simulink model "RLFactoryEnforceCrash6Opponents"  (R2020a)
settings: Solver=VariableStepAuto  StartTime=0.0  StopTime=60  RelTol=1e-3
undefined symbols (not defined in the file): BLOCKEDTIMER, EPS, getRandomSafeCoord, GoalRange, MAXVELOA, MAXVELOB, MAXVELOC, MAXVELOD, MAXVELOE, MAXVELOF, rl, RLStartX, RLStartY, SAFETYDISTANCEA, SAFETYDISTANCEB, SAFETYDISTANCEC, SAFETYDISTANCED, SAFETYDISTANCEE, SAFETYDISTANCEF, THRESHOLDA, THRESHOLDB, THRESHOLDC, THRESHOLDD, THRESHOLDE, THRESHOLDF, TSA, TSB, TSC, TSD, TSE, TSF, TSRL
libraries: rllib x1
(part 2 of 3)

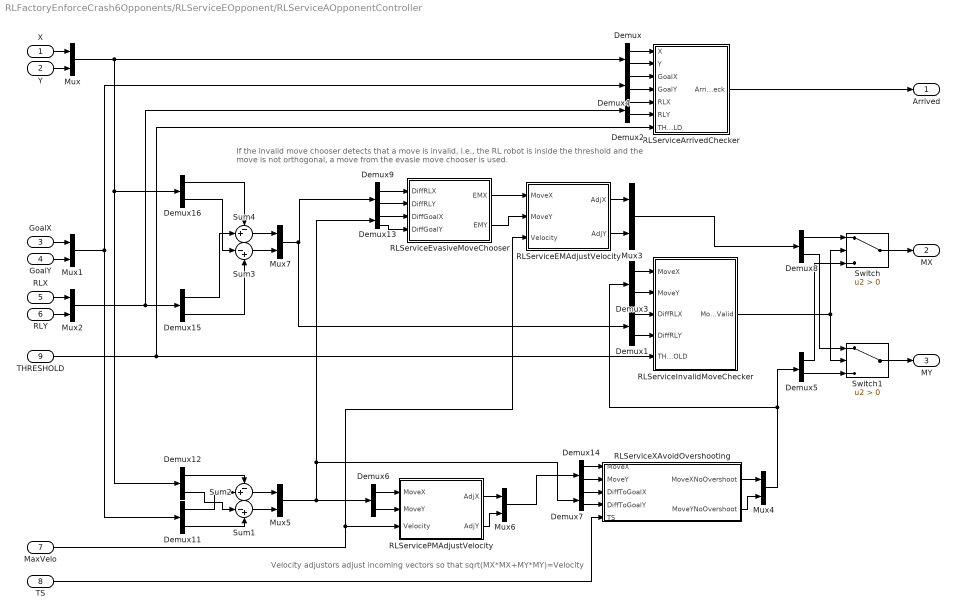
== system RLFactoryEnforceCrash6Opponents/RLServiceEOpponent/RLServiceAOpponentController ==
  note: If the invalid move chooser detects that a move is invalid, i.e.,
      | the RL robot is inside the threshold and the move is not orthogonal, a move from the evasie move chooser is used.
  note: Velocity adjustors adjust incoming vectors so that sqrt(MX*MX+MY*MY)=Velocity
  X : Inport
  Y : Inport  Port=2
  GoalX : Inport  Port=3
  GoalY : Inport  Port=4
  RLX : Inport  Port=5
  RLY : Inport  Port=6
  MaxVelo : Inport  Port=7
  TS : Inport  Port=8
  THRESHOLD : Inport  Port=9
  Demux{,1..9,11..16} (16 alike) : Demux  Outputs=2
  Mux{,1..7} (8 alike) : Mux  Inputs=2
  RLServiceArrivedChecker : Subsystem
  RLServiceEMAdjustVelocity : Subsystem
  RLServiceEvasiveMoveChooser : Subsystem
  RLServiceInvalidMoveChecker : Subsystem
  RLServicePMAdjustVelocity : Subsystem
  RLServiceXAvoidOvershooting : Subsystem
  Sum1 : Sum  Inputs=|-+
  Sum2 : Sum  Inputs=-+|
  Sum3 : Sum  Inputs=|-+
  Sum4 : Sum  Inputs=-+|
  Switch : Switch  Criteria=u2 > Threshold
  Switch1 : Switch  Criteria=u2 > Threshold
  Arrived : Outport
  MX : Outport  Port=2
  MY : Outport  Port=3
  wires:
  GoalX/1 -> Mux1/1
  GoalY/1 -> Mux1/2
  RLServiceArrivedChecker/1(ArrivedCheck) -> Arrived/1
  Demux/1 -> RLServiceArrivedChecker/1(X)
  Demux/2 -> RLServiceArrivedChecker/2(Y)
  Demux4/1 -> RLServiceArrivedChecker/3(GoalX)
  Demux4/2 -> RLServiceArrivedChecker/4(GoalY)
  X/1 -> Mux/1
  Y/1 -> Mux/2
  RLX/1 -> Mux2/1
  RLY/1 -> Mux2/2
  Demux3/1 -> RLServiceInvalidMoveChecker/1(MoveX)
  Demux8/1 -> Switch/1
  Demux5/2 -> Switch1/3
  Demux8/2 -> Switch1/1
  THRESHOLD/1 -> RLServiceArrivedChecker/7(THRESHOLD), RLServiceInvalidMoveChecker/5(THRESHOLD)
  Demux3/2 -> RLServiceInvalidMoveChecker/2(MoveY)
  Demux5/1 -> Switch/3
  RLServiceInvalidMoveChecker/1(MoveInValid) -> Switch/2, Switch1/2
  Switch/1 -> MX/1
  Switch1/1 -> MY/1
  Mux5/1 -> Demux6/1, Demux7/1, Demux13/1
  Demux6/2 -> RLServicePMAdjustVelocity/2(MoveY)
  Mux1/1 -> Demux4/1, Demux11/1
  TS/1 -> RLServiceXAvoidOvershooting/5(TS)
  MaxVelo/1 -> RLServiceEMAdjustVelocity/3(Velocity), RLServicePMAdjustVelocity/3(Velocity)
  RLServicePMAdjustVelocity/1(AdjX) -> Mux6/1
  RLServicePMAdjustVelocity/2(AdjY) -> Mux6/2
  RLServiceEvasiveMoveChooser/1(EMX) -> RLServiceEMAdjustVelocity/1(MoveX)
  RLServiceEvasiveMoveChooser/2(EMY) -> RLServiceEMAdjustVelocity/2(MoveY)
  RLServiceEMAdjustVelocity/1(AdjX) -> Mux3/1
  RLServiceEMAdjustVelocity/2(AdjY) -> Mux3/2
  Mux3/1 -> Demux8/1
  RLServiceXAvoidOvershooting/1(MoveXNoOvershoot) -> Mux4/1
  RLServiceXAvoidOvershooting/2(MoveYNoOvershoot) -> Mux4/2
  Mux4/1 -> Demux5/1, Demux3/1
  Sum2/1 -> Mux5/1
  Sum1/1 -> Mux5/2
  Demux6/1 -> RLServicePMAdjustVelocity/1(MoveX)
  Demux7/1 -> RLServiceXAvoidOvershooting/3(DiffToGoalX)
  Demux7/2 -> RLServiceXAvoidOvershooting/4(DiffToGoalY)
  Demux13/1 -> RLServiceEvasiveMoveChooser/3(DiffGoalX)
  Demux13/2 -> RLServiceEvasiveMoveChooser/4(DiffGoalY)
  Demux11/1 -> Sum2/2
  Demux12/2 -> Sum1/1
  Demux11/2 -> Sum1/2
  Demux12/1 -> Sum2/1
  Demux14/1 -> RLServiceXAvoidOvershooting/1(MoveX)
  Demux14/2 -> RLServiceXAvoidOvershooting/2(MoveY)
  Mux6/1 -> Demux14/1
  Sum3/1 -> Mux7/2
  Demux16/1 -> Sum4/1
  Sum4/1 -> Mux7/1
  Mux/1 -> Demux12/1, Demux16/1, Demux/1
  Mux2/1 -> Demux2/1, Demux15/1
  Demux15/2 -> Sum3/2
  Demux15/1 -> Sum4/2
  Demux16/2 -> Sum3/1
  Demux9/1 -> RLServiceEvasiveMoveChooser/1(DiffRLX)
  Demux9/2 -> RLServiceEvasiveMoveChooser/2(DiffRLY)
  Mux7/1 -> Demux1/1, Demux9/1
  Demux1/1 -> RLServiceInvalidMoveChecker/3(DiffRLX)
  Demux1/2 -> RLServiceInvalidMoveChecker/4(DiffRLY)
  Demux2/2 -> RLServiceArrivedChecker/6(RLY)
  Demux2/1 -> RLServiceArrivedChecker/5(RLX)

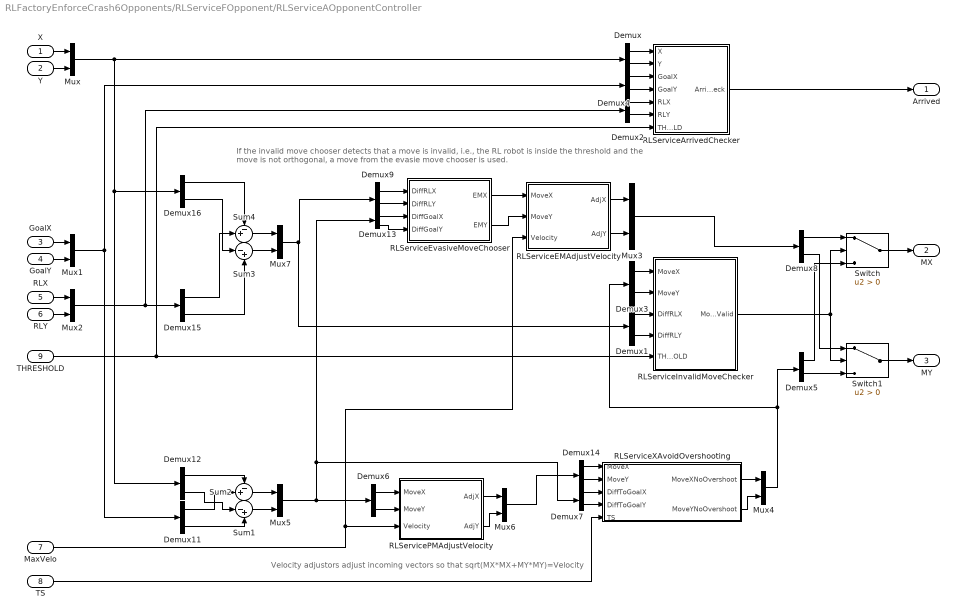
== system RLFactoryEnforceCrash6Opponents/RLServiceFOpponent/RLServiceAOpponentController ==
  note: If the invalid move chooser detects that a move is invalid, i.e.,
      | the RL robot is inside the threshold and the move is not orthogonal, a move from the evasie move chooser is used.
  note: Velocity adjustors adjust incoming vectors so that sqrt(MX*MX+MY*MY)=Velocity
  X : Inport
  Y : Inport  Port=2
  GoalX : Inport  Port=3
  GoalY : Inport  Port=4
  RLX : Inport  Port=5
  RLY : Inport  Port=6
  MaxVelo : Inport  Port=7
  TS : Inport  Port=8
  THRESHOLD : Inport  Port=9
  Demux{,1..9,11..16} (16 alike) : Demux  Outputs=2
  Mux{,1..7} (8 alike) : Mux  Inputs=2
  RLServiceArrivedChecker : Subsystem
  RLServiceEMAdjustVelocity : Subsystem
  RLServiceEvasiveMoveChooser : Subsystem
  RLServiceInvalidMoveChecker : Subsystem
  RLServicePMAdjustVelocity : Subsystem
  RLServiceXAvoidOvershooting : Subsystem
  Sum1 : Sum  Inputs=|-+
  Sum2 : Sum  Inputs=-+|
  Sum3 : Sum  Inputs=|-+
  Sum4 : Sum  Inputs=-+|
  Switch : Switch  Criteria=u2 > Threshold
  Switch1 : Switch  Criteria=u2 > Threshold
  Arrived : Outport
  MX : Outport  Port=2
  MY : Outport  Port=3
  wires:
  GoalX/1 -> Mux1/1
  GoalY/1 -> Mux1/2
  RLServiceArrivedChecker/1(ArrivedCheck) -> Arrived/1
  Demux/1 -> RLServiceArrivedChecker/1(X)
  Demux/2 -> RLServiceArrivedChecker/2(Y)
  Demux4/1 -> RLServiceArrivedChecker/3(GoalX)
  Demux4/2 -> RLServiceArrivedChecker/4(GoalY)
  X/1 -> Mux/1
  Y/1 -> Mux/2
  RLX/1 -> Mux2/1
  RLY/1 -> Mux2/2
  Demux3/1 -> RLServiceInvalidMoveChecker/1(MoveX)
  Demux8/1 -> Switch/1
  Demux5/2 -> Switch1/3
  Demux8/2 -> Switch1/1
  THRESHOLD/1 -> RLServiceArrivedChecker/7(THRESHOLD), RLServiceInvalidMoveChecker/5(THRESHOLD)
  Demux3/2 -> RLServiceInvalidMoveChecker/2(MoveY)
  Demux5/1 -> Switch/3
  RLServiceInvalidMoveChecker/1(MoveInValid) -> Switch/2, Switch1/2
  Switch/1 -> MX/1
  Switch1/1 -> MY/1
  Mux5/1 -> Demux6/1, Demux7/1, Demux13/1
  Demux6/2 -> RLServicePMAdjustVelocity/2(MoveY)
  Mux1/1 -> Demux4/1, Demux11/1
  TS/1 -> RLServiceXAvoidOvershooting/5(TS)
  MaxVelo/1 -> RLServiceEMAdjustVelocity/3(Velocity), RLServicePMAdjustVelocity/3(Velocity)
  RLServicePMAdjustVelocity/1(AdjX) -> Mux6/1
  RLServicePMAdjustVelocity/2(AdjY) -> Mux6/2
  RLServiceEvasiveMoveChooser/1(EMX) -> RLServiceEMAdjustVelocity/1(MoveX)
  RLServiceEvasiveMoveChooser/2(EMY) -> RLServiceEMAdjustVelocity/2(MoveY)
  RLServiceEMAdjustVelocity/1(AdjX) -> Mux3/1
  RLServiceEMAdjustVelocity/2(AdjY) -> Mux3/2
  Mux3/1 -> Demux8/1
  RLServiceXAvoidOvershooting/1(MoveXNoOvershoot) -> Mux4/1
  RLServiceXAvoidOvershooting/2(MoveYNoOvershoot) -> Mux4/2
  Mux4/1 -> Demux5/1, Demux3/1
  Sum2/1 -> Mux5/1
  Sum1/1 -> Mux5/2
  Demux6/1 -> RLServicePMAdjustVelocity/1(MoveX)
  Demux7/1 -> RLServiceXAvoidOvershooting/3(DiffToGoalX)
  Demux7/2 -> RLServiceXAvoidOvershooting/4(DiffToGoalY)
  Demux13/1 -> RLServiceEvasiveMoveChooser/3(DiffGoalX)
  Demux13/2 -> RLServiceEvasiveMoveChooser/4(DiffGoalY)
  Demux11/1 -> Sum2/2
  Demux12/2 -> Sum1/1
  Demux11/2 -> Sum1/2
  Demux12/1 -> Sum2/1
  Demux14/1 -> RLServiceXAvoidOvershooting/1(MoveX)
  Demux14/2 -> RLServiceXAvoidOvershooting/2(MoveY)
  Mux6/1 -> Demux14/1
  Sum3/1 -> Mux7/2
  Demux16/1 -> Sum4/1
  Sum4/1 -> Mux7/1
  Mux/1 -> Demux12/1, Demux16/1, Demux/1
  Mux2/1 -> Demux2/1, Demux15/1
  Demux15/2 -> Sum3/2
  Demux15/1 -> Sum4/2
  Demux16/2 -> Sum3/1
  Demux9/1 -> RLServiceEvasiveMoveChooser/1(DiffRLX)
  Demux9/2 -> RLServiceEvasiveMoveChooser/2(DiffRLY)
  Mux7/1 -> Demux1/1, Demux9/1
  Demux1/1 -> RLServiceInvalidMoveChecker/3(DiffRLX)
  Demux1/2 -> RLServiceInvalidMoveChecker/4(DiffRLY)
  Demux2/2 -> RLServiceArrivedChecker/6(RLY)
  Demux2/1 -> RLServiceArrivedChecker/5(RLX)

== system RLFactoryEnforceCrash6Opponents/RLService6RLRobot/RLService6RLRobotSensor/RLServiceARobotSensorSubsystem ==
  X : Inport
  Y : Inport  Port=2
  OppX : Inport  Port=3
  OppY : Inport  Port=4
  Demux4 : Demux  Outputs=2
  Demux6 : Demux  Outputs=2
  Mux : Mux  Inputs=2
  Mux1 : Mux  Inputs=2
  RLServiceDirectionCalculator : Subsystem
  Sum : Sum  Inputs=-+|
  DiffOppX : Outport
  DiffOppY : Outport  Port=2
  DirOppX : Outport  Port=3
  DirOppY : Outport  Port=4
  wires:
  Mux/1 -> Sum/2, Demux6/1
  Demux6/2 -> RLServiceDirectionCalculator/2(OppY)
  OppX/1 -> Mux/1
  X/1 -> Mux1/1
  Y/1 -> Mux1/2
  Demux6/1 -> RLServiceDirectionCalculator/1(OppX)
  RLServiceDirectionCalculator/1(DirOppX) -> DirOppX/1
  OppY/1 -> Mux/2
  Mux1/1 -> Sum/1
  Sum/1 -> Demux4/1
  RLServiceDirectionCalculator/2(DirOppY) -> DirOppY/1
  Demux4/1 -> DiffOppX/1
  Demux4/2 -> DiffOppY/1

== system RLFactoryEnforceCrash6Opponents/RLService6RLRobot/RLService6RLRobotSensor/RLServiceBRobotSensorSubsystem ==
  X : Inport
  Y : Inport  Port=2
  OppX : Inport  Port=3
  OppY : Inport  Port=4
  Demux4 : Demux  Outputs=2
  Demux6 : Demux  Outputs=2
  Mux : Mux  Inputs=2
  Mux1 : Mux  Inputs=2
  RLServiceDirectionCalculator : Subsystem
  Sum : Sum  Inputs=-+|
  DiffOppX : Outport
  DiffOppY : Outport  Port=2
  DirOppX : Outport  Port=3
  DirOppY : Outport  Port=4
  wires:
  Mux/1 -> Sum/2, Demux6/1
  Demux6/2 -> RLServiceDirectionCalculator/2(OppY)
  OppX/1 -> Mux/1
  X/1 -> Mux1/1
  Y/1 -> Mux1/2
  Demux6/1 -> RLServiceDirectionCalculator/1(OppX)
  RLServiceDirectionCalculator/1(DirOppX) -> DirOppX/1
  OppY/1 -> Mux/2
  Mux1/1 -> Sum/1
  Sum/1 -> Demux4/1
  RLServiceDirectionCalculator/2(DirOppY) -> DirOppY/1
  Demux4/1 -> DiffOppX/1
  Demux4/2 -> DiffOppY/1

== system RLFactoryEnforceCrash6Opponents/RLService6RLRobot/RLService6RLRobotSensor/RLServiceCRobotSensorSubsystem ==
  X : Inport
  Y : Inport  Port=2
  OppX : Inport  Port=3
  OppY : Inport  Port=4
  Demux4 : Demux  Outputs=2
  Demux6 : Demux  Outputs=2
  Mux : Mux  Inputs=2
  Mux1 : Mux  Inputs=2
  RLServiceDirectionCalculator : Subsystem
  Sum : Sum  Inputs=-+|
  DiffOppX : Outport
  DiffOppY : Outport  Port=2
  DirOppX : Outport  Port=3
  DirOppY : Outport  Port=4
  wires:
  Mux/1 -> Sum/2, Demux6/1
  Demux6/2 -> RLServiceDirectionCalculator/2(OppY)
  OppX/1 -> Mux/1
  X/1 -> Mux1/1
  Y/1 -> Mux1/2
  Demux6/1 -> RLServiceDirectionCalculator/1(OppX)
  RLServiceDirectionCalculator/1(DirOppX) -> DirOppX/1
  OppY/1 -> Mux/2
  Mux1/1 -> Sum/1
  Sum/1 -> Demux4/1
  RLServiceDirectionCalculator/2(DirOppY) -> DirOppY/1
  Demux4/1 -> DiffOppX/1
  Demux4/2 -> DiffOppY/1

== system RLFactoryEnforceCrash6Opponents/RLService6RLRobot/RLService6RLRobotSensor/RLServiceDRobotSensorSubsystem ==
  X : Inport
  Y : Inport  Port=2
  OppX : Inport  Port=3
  OppY : Inport  Port=4
  Demux4 : Demux  Outputs=2
  Demux6 : Demux  Outputs=2
  Mux : Mux  Inputs=2
  Mux1 : Mux  Inputs=2
  RLServiceDirectionCalculator : Subsystem
  Sum : Sum  Inputs=-+|
  DiffOppX : Outport
  DiffOppY : Outport  Port=2
  DirOppX : Outport  Port=3
  DirOppY : Outport  Port=4
  wires:
  Mux/1 -> Sum/2, Demux6/1
  Demux6/2 -> RLServiceDirectionCalculator/2(OppY)
  OppX/1 -> Mux/1
  X/1 -> Mux1/1
  Y/1 -> Mux1/2
  Demux6/1 -> RLServiceDirectionCalculator/1(OppX)
  RLServiceDirectionCalculator/1(DirOppX) -> DirOppX/1
  OppY/1 -> Mux/2
  Mux1/1 -> Sum/1
  Sum/1 -> Demux4/1
  RLServiceDirectionCalculator/2(DirOppY) -> DirOppY/1
  Demux4/1 -> DiffOppX/1
  Demux4/2 -> DiffOppY/1

== system RLFactoryEnforceCrash6Opponents/RLService6RLRobot/RLService6RLRobotSensor/RLServiceERobotSensorSubsystem ==
  X : Inport
  Y : Inport  Port=2
  OppX : Inport  Port=3
  OppY : Inport  Port=4
  Demux4 : Demux  Outputs=2
  Demux6 : Demux  Outputs=2
  Mux : Mux  Inputs=2
  Mux1 : Mux  Inputs=2
  RLServiceDirectionCalculator : Subsystem
  Sum : Sum  Inputs=-+|
  DiffOppX : Outport
  DiffOppY : Outport  Port=2
  DirOppX : Outport  Port=3
  DirOppY : Outport  Port=4
  wires:
  Mux/1 -> Sum/2, Demux6/1
  Demux6/2 -> RLServiceDirectionCalculator/2(OppY)
  OppX/1 -> Mux/1
  X/1 -> Mux1/1
  Y/1 -> Mux1/2
  Demux6/1 -> RLServiceDirectionCalculator/1(OppX)
  RLServiceDirectionCalculator/1(DirOppX) -> DirOppX/1
  OppY/1 -> Mux/2
  Mux1/1 -> Sum/1
  Sum/1 -> Demux4/1
  RLServiceDirectionCalculator/2(DirOppY) -> DirOppY/1
  Demux4/1 -> DiffOppX/1
  Demux4/2 -> DiffOppY/1

== system RLFactoryEnforceCrash6Opponents/RLService6RLRobot/RLService6RLRobotSensor/RLServiceFRobotSensorSubsystem ==
  X : Inport
  Y : Inport  Port=2
  OppX : Inport  Port=3
  OppY : Inport  Port=4
  Demux4 : Demux  Outputs=2
  Demux6 : Demux  Outputs=2
  Mux : Mux  Inputs=2
  Mux1 : Mux  Inputs=2
  RLServiceDirectionCalculator : Subsystem
  Sum : Sum  Inputs=-+|
  DiffOppX : Outport
  DiffOppY : Outport  Port=2
  DirOppX : Outport  Port=3
  DirOppY : Outport  Port=4
  wires:
  Mux/1 -> Sum/2, Demux6/1
  Demux6/2 -> RLServiceDirectionCalculator/2(OppY)
  OppX/1 -> Mux/1
  X/1 -> Mux1/1
  Y/1 -> Mux1/2
  Demux6/1 -> RLServiceDirectionCalculator/1(OppX)
  RLServiceDirectionCalculator/1(DirOppX) -> DirOppX/1
  OppY/1 -> Mux/2
  Mux1/1 -> Sum/1
  Sum/1 -> Demux4/1
  RLServiceDirectionCalculator/2(DirOppY) -> DirOppY/1
  Demux4/1 -> DiffOppX/1
  Demux4/2 -> DiffOppY/1

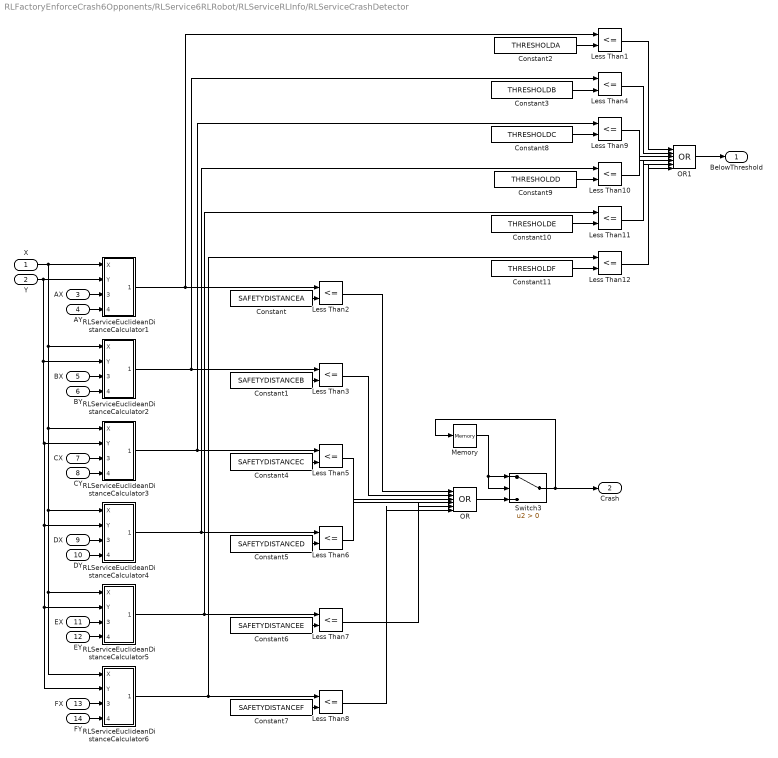
== system RLFactoryEnforceCrash6Opponents/RLService6RLRobot/RLServiceRLInfo/RLServiceCrashDetector ==
  X : Inport
  Y : Inport  Port=2
  AX : Inport  Port=3
  AY : Inport  Port=4
  BX : Inport  Port=5
  BY : Inport  Port=6
  CX : Inport  Port=7
  CY : Inport  Port=8
  DX : Inport  Port=9
  DY : Inport  Port=10
  EX : Inport  Port=11
  EY : Inport  Port=12
  FX : Inport  Port=13
  FY : Inport  Port=14
  Constant : Constant  Value=SAFETYDISTANCEA
  Constant1 : Constant  Value=SAFETYDISTANCEB
  Constant10 : Constant  Value=THRESHOLDE
  Constant11 : Constant  Value=THRESHOLDF
  Constant2 : Constant  Value=THRESHOLDA
  Constant3 : Constant  Value=THRESHOLDB
  Constant4 : Constant  Value=SAFETYDISTANCEC
  Constant5 : Constant  Value=SAFETYDISTANCED
  Constant6 : Constant  Value=SAFETYDISTANCEE
  Constant7 : Constant  Value=SAFETYDISTANCEF
  Constant8 : Constant  Value=THRESHOLDC
  Constant9 : Constant  Value=THRESHOLDD
  Less Than{1..12} (12 alike) : RelationalOperator  Operator=<=  OutDataTypeStr=boolean  RndMeth=Simplest
  Memory : Memory
  OR : Logic  Operator=OR  Inputs=6  IconShape=distinctive  AllPortsSameDT=off  OutDataTypeStr=boolean
  OR1 : Logic  Operator=OR  Inputs=6  IconShape=distinctive  AllPortsSameDT=off  OutDataTypeStr=boolean
  RLServiceEuclideanDistanceCalculator1 : Subsystem
  RLServiceEuclideanDistanceCalculator2 : Subsystem
  RLServiceEuclideanDistanceCalculator3 : Subsystem
  RLServiceEuclideanDistanceCalculator4 : Subsystem
  RLServiceEuclideanDistanceCalculator5 : Subsystem
  RLServiceEuclideanDistanceCalculator6 : Subsystem
  Switch3 : Switch  Criteria=u2 > Threshold
  BelowThreshold : Outport
  Crash : Outport  Port=2
  wires:
  AX/1 -> RLServiceEuclideanDistanceCalculator1/3(XOpp)
  Less Than2/1 -> OR/1
  Memory/1 -> Switch3/2, Switch3/1
  Constant/1 -> Less Than2/2
  AY/1 -> RLServiceEuclideanDistanceCalculator1/4(YOpp)
  OR/1 -> Switch3/3
  Constant1/1 -> Less Than3/2
  BY/1 -> RLServiceEuclideanDistanceCalculator2/4(YOpp)
  Less Than3/1 -> OR/2
  BX/1 -> RLServiceEuclideanDistanceCalculator2/3(XOpp)
  Switch3/1 -> Crash/1, Memory/1
  Constant2/1 -> Less Than1/2
  RLServiceEuclideanDistanceCalculator1/1(Dist) -> Less Than2/1, Less Than1/1
  Constant3/1 -> Less Than4/2
  RLServiceEuclideanDistanceCalculator2/1(Dist) -> Less Than4/1, Less Than3/1
  Less Than1/1 -> OR1/1
  Less Than4/1 -> OR1/2
  OR1/1 -> BelowThreshold/1
  DY/1 -> RLServiceEuclideanDistanceCalculator4/4(YOpp)
  Less Than5/1 -> OR/3
  Constant5/1 -> Less Than6/2
  Constant4/1 -> Less Than5/2
  RLServiceEuclideanDistanceCalculator3/1(Dist) -> Less Than9/1, Less Than5/1
  Less Than6/1 -> OR/4
  DX/1 -> RLServiceEuclideanDistanceCalculator4/3(XOpp)
  CX/1 -> RLServiceEuclideanDistanceCalculator3/3(XOpp)
  RLServiceEuclideanDistanceCalculator4/1(Dist) -> Less Than10/1, Less Than6/1
  CY/1 -> RLServiceEuclideanDistanceCalculator3/4(YOpp)
  EX/1 -> RLServiceEuclideanDistanceCalculator5/3(XOpp)
  EY/1 -> RLServiceEuclideanDistanceCalculator5/4(YOpp)
  RLServiceEuclideanDistanceCalculator5/1(Dist) -> Less Than7/1, Less Than11/1
  Constant6/1 -> Less Than7/2
  FY/1 -> RLServiceEuclideanDistanceCalculator6/4(YOpp)
  Constant7/1 -> Less Than8/2
  Y/1 -> RLServiceEuclideanDistanceCalculator6/2(Y), RLServiceEuclideanDistanceCalculator5/2(Y), RLServiceEuclideanDistanceCalculator4/2(Y), RLServiceEuclideanDistanceCalculator3/2(Y), RLServiceEuclideanDistanceCalculator2/2(Y), RLServiceEuclideanDistanceCalculator1/2(Y)
  X/1 -> RLServiceEuclideanDistanceCalculator1/1(X), RLServiceEuclideanDistanceCalculator6/1(X), RLServiceEuclideanDistanceCalculator5/1(X), RLServiceEuclideanDistanceCalculator4/1(X), RLServiceEuclideanDistanceCalculator3/1(X), RLServiceEuclideanDistanceCalculator2/1(X)
  FX/1 -> RLServiceEuclideanDistanceCalculator6/3(XOpp)
  RLServiceEuclideanDistanceCalculator6/1(Dist) -> Less Than8/1, Less Than12/1
  Less Than7/1 -> OR/5
  Less Than8/1 -> OR/6
  Constant8/1 -> Less Than9/2
  Less Than9/1 -> OR1/3
  Less Than11/1 -> OR1/5
  Less Than10/1 -> OR1/4
  Constant10/1 -> Less Than11/2
  Constant9/1 -> Less Than10/2
  Less Than12/1 -> OR1/6
  Constant11/1 -> Less Than12/2

== system RLFactoryEnforceCrash6Opponents/RLService6RLRobot/RLServiceRLInfo/RLServiceGoalTracker ==
  X : Inport
  Y : Inport  Port=2
  GoalX : Inport  Port=3
  GoalY : Inport  Port=4
  Constant1 : Constant
  Constant5 : Constant  Value=0.5
  Constant7 : Constant  Value=0
  Less Than1 : RelationalOperator  Operator=<  OutDataTypeStr=boolean  RndMeth=Simplest
  RLServiceEuclideanDistanceCalculator : Subsystem
  Switch : Switch  Criteria=u2 > Threshold
  Dist : Outport
  Arrived : Outport  Port=2
  wires:
  Constant7/1 -> Switch/3
  GoalX/1 -> RLServiceEuclideanDistanceCalculator/3(GoalX)
  Y/1 -> RLServiceEuclideanDistanceCalculator/2(Y)
  RLServiceEuclideanDistanceCalculator/1(DistGoal) -> Dist/1, Less Than1/1
  Constant1/1 -> Switch/1
  Switch/1 -> Arrived/1
  Less Than1/1 -> Switch/2
  X/1 -> RLServiceEuclideanDistanceCalculator/1(X)
  GoalY/1 -> RLServiceEuclideanDistanceCalculator/4(GoalY)
  Constant5/1 -> Less Than1/2

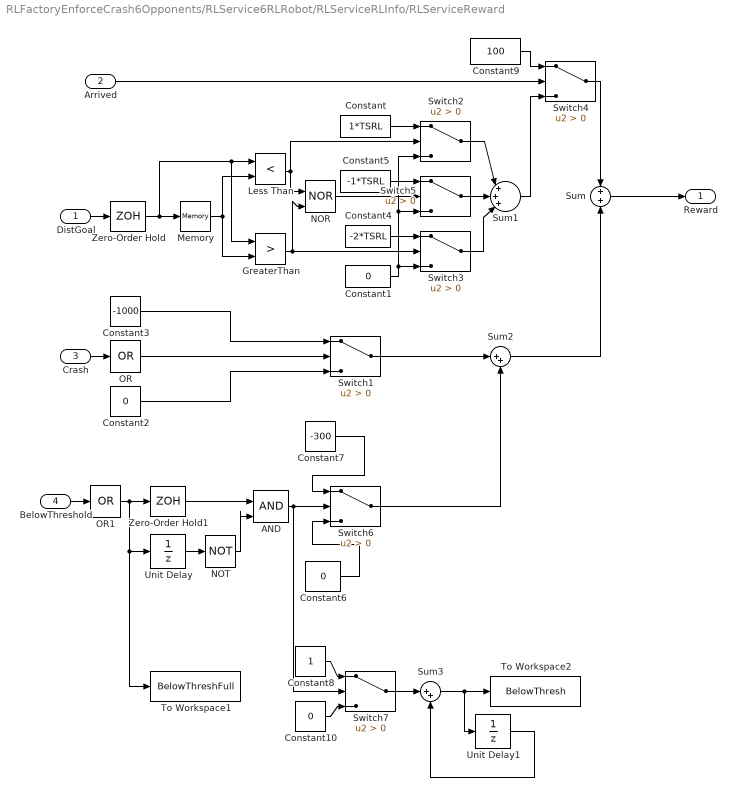
== system RLFactoryEnforceCrash6Opponents/RLService6RLRobot/RLServiceRLInfo/RLServiceReward ==
  DistGoal : Inport
  Arrived : Inport  Port=2
  Crash : Inport  Port=3
  BelowThreshold : Inport  Port=4
  AND : Logic  IconShape=distinctive  AllPortsSameDT=off  OutDataTypeStr=boolean
  Constant : Constant  Value=1*TSRL
  Constant{1..2,6,10} (4 alike) : Constant  Value=0
  Constant3 : Constant  Value=-1000  VectorParams1D=off
  Constant4 : Constant  Value=-2*TSRL
  Constant5 : Constant  Value=-1*TSRL
  Constant7 : Constant  Value=-300  VectorParams1D=off
  Constant8 : Constant
  Constant9 : Constant  Value=100
  GreaterThan : RelationalOperator  Operator=>  OutDataTypeStr=boolean  RndMeth=Simplest
  Less Than : RelationalOperator  Operator=<  OutDataTypeStr=boolean  RndMeth=Simplest
  Memory : Memory
  NOR : Logic  Operator=NOR  IconShape=distinctive  AllPortsSameDT=off  OutDataTypeStr=boolean
  NOT : Logic  Operator=NOT  IconShape=distinctive  AllPortsSameDT=off  OutDataTypeStr=boolean
  OR : Logic  Operator=OR  Inputs=1  IconShape=distinctive  AllPortsSameDT=off  OutDataTypeStr=boolean
  OR1 : Logic  Operator=OR  Inputs=1  IconShape=distinctive  AllPortsSameDT=off  OutDataTypeStr=boolean
  Sum : Sum
  Sum1 : Sum  Inputs=|+++|
  Sum2 : Sum  Inputs=|++
  Sum3 : Sum  Inputs=|++
  Switch{1..7} (7 alike) : Switch  Criteria=u2 > Threshold
  To Workspace1 : ToWorkspace  VariableName=BelowThreshFull  SampleTime=TSRL
  To Workspace2 : ToWorkspace  VariableName=BelowThresh  SampleTime=TSRL
      settings: MaxDataPoints=1
  Unit Delay : UnitDelay  SampleTime=TSRL  HasFrameUpgradeWarning=on
  Unit Delay1 : UnitDelay  SampleTime=TSRL  HasFrameUpgradeWarning=on
  Zero-Order Hold : ZeroOrderHold  SampleTime=TSRL
  Zero-Order Hold1 : ZeroOrderHold  SampleTime=TSRL
  Reward : Outport
  wires:
  Sum/1 -> Reward/1
  Constant2/1 -> Switch1/3
  Constant3/1 -> Switch1/1
  Sum2/1 -> Sum/2
  DistGoal/1 -> Zero-Order Hold/1
  Memory/1 -> GreaterThan/2, Less Than/2
  Switch4/1 -> Sum/1
  Constant9/1 -> Switch4/1
  Switch2/1 -> Sum1/1
  Arrived/1 -> Switch4/2
  OR/1 -> Switch1/2
  Less Than/1 -> NOR/1, Switch2/2
  Constant/1 -> Switch2/1
  Constant1/1 -> Switch2/3, Switch5/3, Switch3/3
  GreaterThan/1 -> NOR/2, Switch3/2
  Constant4/1 -> Switch3/1
  Sum1/1 -> Switch4/3
  Switch3/1 -> Sum1/3
  NOR/1 -> Switch5/2
  Constant5/1 -> Switch5/1
  Switch5/1 -> Sum1/2
  Zero-Order Hold/1 -> Memory/1, GreaterThan/1, Less Than/1
  Crash/1 -> OR/1
  OR1/1 -> Zero-Order Hold1/1, To Workspace1/1, Unit Delay/1
  Constant7/1 -> Switch6/1
  BelowThreshold/1 -> OR1/1
  Constant6/1 -> Switch6/3
  Switch6/1 -> Sum2/2
  Switch1/1 -> Sum2/1
  Unit Delay/1 -> NOT/1
  NOT/1 -> AND/2
  Sum3/1 -> To Workspace2/1, Unit Delay1/1
  Zero-Order Hold1/1 -> AND/1
  Unit Delay1/1 -> Sum3/2
  Switch7/1 -> Sum3/1
  Constant8/1 -> Switch7/1
  Constant10/1 -> Switch7/3
  AND/1 -> Switch7/2, Switch6/2

== system RLFactoryEnforceCrash6Opponents/RLService6RLRobot/RLServiceRLMotorControl/RLServiceRLAdjustVelocity ==
  MoveX : Inport
  MoveY : Inport  Port=2
  Velocity : Inport  Port=3
  Constant : Constant
  Demux1 : Demux  Outputs=2
  Divide : Product  Inputs=*/
  Divide1 : Product  Inputs=*/
  Mux : Mux  Inputs=2
  Product : Product
  Product3 : Product
  Sqrt1 : Sqrt  SaturateOnIntegerOverflow=on
  Square : Math  Operator=square  SaturateOnIntegerOverflow=on
  Square1 : Math  Operator=square  SaturateOnIntegerOverflow=on
  Sum : Sum  Inputs=+|+
  Switch : Switch  Criteria=u2 > Threshold
  AdjMX : Outport
  AdjMY : Outport  Port=2
  wires:
  Product/1 -> AdjMX/1
  MoveY/1 -> Square1/1, Mux/2
  Mux/1 -> Demux1/1
  Divide1/1 -> Product3/1
  Constant/1 -> Switch/3
  Square1/1 -> Sum/2
  Switch/1 -> Divide1/2, Divide/2
  Velocity/1 -> Product/2, Product3/2
  Sum/1 -> Sqrt1/1
  Square/1 -> Sum/1
  Sqrt1/1 -> Switch/2, Switch/1
  Product3/1 -> AdjMY/1
  Demux1/2 -> Divide1/1
  MoveX/1 -> Square/1, Mux/1
  Demux1/1 -> Divide/1
  Divide/1 -> Product/1

== system RLFactoryEnforceCrash6Opponents/RLServiceAOpponent/RLServiceAOpponentController/RLServiceArrivedChecker ==
  X : Inport
  Y : Inport  Port=2
  GoalX : Inport  Port=3
  GoalY : Inport  Port=4
  RLX : Inport  Port=5
  RLY : Inport  Port=6
  THRESHOLD : Inport  Port=7
  Constant1 : Constant
  Constant3 : Constant
  Constant4 : Constant  Value=0
  Constant5 : Constant  Value=0
  Constant6 : Constant
  Constant8 : Constant  Value=-BLOCKEDTIMER
  Integrator : Integrator  LimitOutput=on  UpperSaturationLimit=BLOCKEDTIMER  LowerSaturationLimit=0
  RLServiceEuclideanDistanceCalculator1 : Subsystem
  RLServiceEuclideanDistanceCalculator2 : Subsystem
  Sum : Sum  Inputs=|++
  Sum1 : Sum  Inputs=+-|
  Switch1 : Switch  Criteria=u2 > Threshold  Threshold=0.5
  Switch3 : Switch  Threshold=BLOCKEDTIMER
  Switch4 : Switch  Criteria=u2 > Threshold
  ArrivedCheck : Outport
  wires:
  RLServiceEuclideanDistanceCalculator1/1(DistToGoal) -> Switch1/2
  X/1 -> RLServiceEuclideanDistanceCalculator1/1(X)
  Switch1/1 -> Sum/1
  Constant3/1 -> Switch1/3
  Y/1 -> RLServiceEuclideanDistanceCalculator1/2(Y)
  Constant4/1 -> Switch1/1
  Sum/1 -> ArrivedCheck/1
  Switch3/1 -> Sum/2
  Integrator/1 -> Switch3/2
  Constant5/1 -> Switch3/3
  RLX/1 -> RLServiceEuclideanDistanceCalculator2/1(X)
  RLY/1 -> RLServiceEuclideanDistanceCalculator2/2(Y)
  GoalX/1 -> RLServiceEuclideanDistanceCalculator2/3(GoalX), RLServiceEuclideanDistanceCalculator1/3(GoalX)
  GoalY/1 -> RLServiceEuclideanDistanceCalculator2/4(GoalY), RLServiceEuclideanDistanceCalculator1/4(GoalY)
  RLServiceEuclideanDistanceCalculator2/1(OppDistToGoal) -> Sum1/1
  Constant8/1 -> Switch4/1
  Constant6/1 -> Switch4/3
  THRESHOLD/1 -> Sum1/2
  Sum1/1 -> Switch4/2
  Switch4/1 -> Integrator/1
  Constant1/1 -> Switch3/1

== system RLFactoryEnforceCrash6Opponents/RLServiceAOpponent/RLServiceAOpponentController/RLServiceEMAdjustVelocity ==
  MoveX : Inport
  MoveY : Inport  Port=2
  Velocity : Inport  Port=3
  Constant : Constant
  Demux1 : Demux  Outputs=2
  Divide : Product  Inputs=*/
  Divide1 : Product  Inputs=*/
  Mux : Mux  Inputs=2
  Product : Product
  Product3 : Product
  Sqrt1 : Sqrt  SaturateOnIntegerOverflow=on
  Square : Math  Operator=square  SaturateOnIntegerOverflow=on
  Square1 : Math  Operator=square  SaturateOnIntegerOverflow=on
  Sum : Sum  Inputs=+|+
  Switch : Switch  Criteria=u2 > Threshold
  AdjX : Outport
  AdjY : Outport  Port=2
  wires:
  Product/1 -> AdjX/1
  MoveY/1 -> Square1/1, Mux/2
  Mux/1 -> Demux1/1
  Divide1/1 -> Product3/1
  Constant/1 -> Switch/3
  Square1/1 -> Sum/2
  Switch/1 -> Divide1/2, Divide/2
  Velocity/1 -> Product/2, Product3/2
  Sum/1 -> Sqrt1/1
  Square/1 -> Sum/1
  Sqrt1/1 -> Switch/2, Switch/1
  Product3/1 -> AdjY/1
  Demux1/2 -> Divide1/1
  MoveX/1 -> Square/1, Mux/1
  Demux1/1 -> Divide/1
  Divide/1 -> Product/1

== system RLFactoryEnforceCrash6Opponents/RLServiceAOpponent/RLServiceAOpponentController/RLServiceEvasiveMoveChooser ==
  DiffRLX : Inport
  DiffRLY : Inport  Port=2
  DiffGoalX : Inport  Port=3
  DiffGoalY : Inport  Port=4
  Abs : Abs
  Abs1 : Abs
  Demux{,2..4} (4 alike) : Demux  Outputs=2
  Gain : Gain  Gain=-1
  Gain1 : Gain  Gain=-1
  Mux1 : Mux  Inputs=2
  Mux2 : Mux  Inputs=2
  Mux3 : Mux  Inputs=2
  Sqrt : Sqrt  SaturateOnIntegerOverflow=on
  Sqrt1 : Sqrt  SaturateOnIntegerOverflow=on
  Sum{,1..2,5} (4 alike) : Sum  Inputs=+|+
  Sum6 : Sum  Inputs=+|-
  Switch : Switch  Criteria=u2 > Threshold
  Switch1 : Switch  Criteria=u2 > Threshold
  EMX : Outport
  EMY : Outport  Port=2
  wires:
  Gain/1 -> Mux1/1
  DiffRLX/1 -> Gain1/1, Mux1/2
  Gain1/1 -> Mux2/2
  DiffGoalX/1 -> Mux3/1
  DiffGoalY/1 -> Mux3/2
  Mux3/1 -> Sum/2, Sum1/2
  Mux2/1 -> Sum/1, Demux4/1
  Mux1/1 -> Demux3/1, Sum1/1
  Sum1/1 -> Abs/1
  Sum/1 -> Abs1/1
  Abs1/1 -> Demux/1
  Demux/1 -> Sum2/1
  Demux/2 -> Sum2/2
  Demux2/2 -> Sum5/2
  Demux2/1 -> Sum5/1
  Abs/1 -> Demux2/1
  Sum5/1 -> Sqrt/1
  Sum2/1 -> Sqrt1/1
  Sqrt/1 -> Sum6/1
  Sqrt1/1 -> Sum6/2
  Sum6/1 -> Switch/2, Switch1/2
  Demux3/1 -> Switch/1
  Demux3/2 -> Switch1/1
  Demux4/1 -> Switch/3
  Demux4/2 -> Switch1/3
  Switch/1 -> EMX/1
  Switch1/1 -> EMY/1
  DiffRLY/1 -> Mux2/1, Gain/1

== system RLFactoryEnforceCrash6Opponents/RLServiceAOpponent/RLServiceAOpponentController/RLServiceInvalidMoveChecker ==
  MoveX : Inport
  MoveY : Inport  Port=2
  DiffRLX : Inport  Port=3
  DiffRLY : Inport  Port=4
  THRESHOLD : Inport  Port=5
  Constant5 : Constant
  Constant6 : Constant  Value=0
  Constant7 : Constant  Value=0
  Constant8 : Constant
  Constant9 : Constant
  Product : Product
  Product1 : Product
  Square : Math  Operator=square  SaturateOnIntegerOverflow=on
  Square Root : Sqrt  SaturateOnIntegerOverflow=on
  Square1 : Math  Operator=square  SaturateOnIntegerOverflow=on
  Sum : Sum  Inputs=+|-
  Sum1 : Sum
  Sum5 : Sum  Inputs=+|+
  Sum6 : Sum  Inputs=+|-|+
  Switch1 : Switch  Criteria=u2 > Threshold
  Switch3 : Switch  Criteria=u2 > Threshold
  MoveInValid : Outport
  wires:
  Product1/1 -> Sum5/2
  Sum5/1 -> Switch3/2
  Product/1 -> Sum5/1
  Sum6/1 -> MoveInValid/1
  Switch3/1 -> Sum6/1
  Constant9/1 -> Switch3/1
  MoveY/1 -> Product1/1
  MoveX/1 -> Product/1
  Constant8/1 -> Sum6/2
  Constant7/1 -> Switch3/3
  THRESHOLD/1 -> Sum/2
  Sum/1 -> Switch1/2
  Constant5/1 -> Switch1/3
  Constant6/1 -> Switch1/1
  Switch1/1 -> Sum6/3
  DiffRLY/1 -> Square1/1, Product1/2
  DiffRLX/1 -> Product/2, Square/1
  Square1/1 -> Sum1/2
  Sum1/1 -> Square Root/1
  Square/1 -> Sum1/1
  Square Root/1 -> Sum/1

== system RLFactoryEnforceCrash6Opponents/RLServiceAOpponent/RLServiceAOpponentController/RLServicePMAdjustVelocity ==
  MoveX : Inport
  MoveY : Inport  Port=2
  Velocity : Inport  Port=3
  Constant : Constant
  Demux1 : Demux  Outputs=2
  Divide : Product  Inputs=*/
  Divide1 : Product  Inputs=*/
  Mux : Mux  Inputs=2
  Product : Product
  Product3 : Product
  Sqrt1 : Sqrt  SaturateOnIntegerOverflow=on
  Square : Math  Operator=square  SaturateOnIntegerOverflow=on
  Square1 : Math  Operator=square  SaturateOnIntegerOverflow=on
  Sum : Sum  Inputs=+|+
  Switch : Switch  Criteria=u2 > Threshold
  AdjX : Outport
  AdjY : Outport  Port=2
  wires:
  Velocity/1 -> Product/2, Product3/2
  MoveX/1 -> Square/1, Mux/1
  MoveY/1 -> Square1/1, Mux/2
  Divide1/1 -> Product3/1
  Divide/1 -> Product/1
  Switch/1 -> Divide1/2, Divide/2
  Constant/1 -> Switch/3
  Mux/1 -> Demux1/1
  Demux1/2 -> Divide1/1
  Square1/1 -> Sum/2
  Sum/1 -> Sqrt1/1
  Demux1/1 -> Divide/1
  Product/1 -> AdjX/1
  Sqrt1/1 -> Switch/2, Switch/1
  Product3/1 -> AdjY/1
  Square/1 -> Sum/1

== system RLFactoryEnforceCrash6Opponents/RLServiceAOpponent/RLServiceAOpponentController/RLServiceXAvoidOvershooting ==
  MoveX : Inport
  MoveY : Inport  Port=2
  DiffToGoalX : Inport  Port=3
  DiffToGoalY : Inport  Port=4
  TS : Inport  Port=5
  Abs{1..4} (4 alike) : Abs
  Divide : Product  Inputs=*/
  Divide1 : Product  Inputs=*/
  Product : Product
  Product1 : Product
  Sum1 : Sum  Inputs=-|+
  Sum2 : Sum  Inputs=-|+
  Switch : Switch  Criteria=u2 > Threshold
  Switch1 : Switch  Criteria=u2 > Threshold
  MoveXNoOvershoot : Outport
  MoveYNoOvershoot : Outport  Port=2
  wires:
  Abs1/1 -> Sum1/2
  Switch/1 -> MoveXNoOvershoot/1
  Product/1 -> Abs2/1
  Abs2/1 -> Sum1/1
  DiffToGoalX/1 -> Divide/1, Abs1/1
  Sum1/1 -> Switch/2
  MoveX/1 -> Product/1, Switch/1
  Divide/1 -> Switch/3
  MoveY/1 -> Product1/1, Switch1/1
  Sum2/1 -> Switch1/2
  Abs4/1 -> Sum2/1
  Product1/1 -> Abs4/1
  Divide1/1 -> Switch1/3
  TS/1 -> Divide1/2, Product1/2, Divide/2, Product/2
  Abs3/1 -> Sum2/2
  Switch1/1 -> MoveYNoOvershoot/1
  DiffToGoalY/1 -> Divide1/1, Abs3/1

== system RLFactoryEnforceCrash6Opponents/RLServiceBOpponent/RLServiceAOpponentController/RLServiceArrivedChecker ==
  X : Inport
  Y : Inport  Port=2
  GoalX : Inport  Port=3
  GoalY : Inport  Port=4
  RLX : Inport  Port=5
  RLY : Inport  Port=6
  THRESHOLD : Inport  Port=7
  Constant1 : Constant
  Constant3 : Constant
  Constant4 : Constant  Value=0
  Constant5 : Constant  Value=0
  Constant6 : Constant
  Constant8 : Constant  Value=-BLOCKEDTIMER
  Integrator : Integrator  LimitOutput=on  UpperSaturationLimit=BLOCKEDTIMER  LowerSaturationLimit=0
  RLServiceEuclideanDistanceCalculator1 : Subsystem
  RLServiceEuclideanDistanceCalculator2 : Subsystem
  Sum : Sum  Inputs=|++
  Sum1 : Sum  Inputs=+-|
  Switch1 : Switch  Criteria=u2 > Threshold  Threshold=0.5
  Switch3 : Switch  Threshold=BLOCKEDTIMER
  Switch4 : Switch  Criteria=u2 > Threshold
  ArrivedCheck : Outport
  wires:
  RLServiceEuclideanDistanceCalculator1/1(DistToGoal) -> Switch1/2
  X/1 -> RLServiceEuclideanDistanceCalculator1/1(X)
  Switch1/1 -> Sum/1
  Constant3/1 -> Switch1/3
  Y/1 -> RLServiceEuclideanDistanceCalculator1/2(Y)
  Constant4/1 -> Switch1/1
  Sum/1 -> ArrivedCheck/1
  Switch3/1 -> Sum/2
  Integrator/1 -> Switch3/2
  Constant5/1 -> Switch3/3
  RLX/1 -> RLServiceEuclideanDistanceCalculator2/1(X)
  RLY/1 -> RLServiceEuclideanDistanceCalculator2/2(Y)
  GoalX/1 -> RLServiceEuclideanDistanceCalculator2/3(GoalX), RLServiceEuclideanDistanceCalculator1/3(GoalX)
  GoalY/1 -> RLServiceEuclideanDistanceCalculator2/4(GoalY), RLServiceEuclideanDistanceCalculator1/4(GoalY)
  RLServiceEuclideanDistanceCalculator2/1(OppDistToGoal) -> Sum1/1
  Constant8/1 -> Switch4/1
  Constant6/1 -> Switch4/3
  THRESHOLD/1 -> Sum1/2
  Sum1/1 -> Switch4/2
  Switch4/1 -> Integrator/1
  Constant1/1 -> Switch3/1

== system RLFactoryEnforceCrash6Opponents/RLServiceBOpponent/RLServiceAOpponentController/RLServiceEMAdjustVelocity ==
  MoveX : Inport
  MoveY : Inport  Port=2
  Velocity : Inport  Port=3
  Constant : Constant
  Demux1 : Demux  Outputs=2
  Divide : Product  Inputs=*/
  Divide1 : Product  Inputs=*/
  Mux : Mux  Inputs=2
  Product : Product
  Product3 : Product
  Sqrt1 : Sqrt  SaturateOnIntegerOverflow=on
  Square : Math  Operator=square  SaturateOnIntegerOverflow=on
  Square1 : Math  Operator=square  SaturateOnIntegerOverflow=on
  Sum : Sum  Inputs=+|+
  Switch : Switch  Criteria=u2 > Threshold
  AdjX : Outport
  AdjY : Outport  Port=2
  wires:
  Product/1 -> AdjX/1
  MoveY/1 -> Square1/1, Mux/2
  Mux/1 -> Demux1/1
  Divide1/1 -> Product3/1
  Constant/1 -> Switch/3
  Square1/1 -> Sum/2
  Switch/1 -> Divide1/2, Divide/2
  Velocity/1 -> Product/2, Product3/2
  Sum/1 -> Sqrt1/1
  Square/1 -> Sum/1
  Sqrt1/1 -> Switch/2, Switch/1
  Product3/1 -> AdjY/1
  Demux1/2 -> Divide1/1
  MoveX/1 -> Square/1, Mux/1
  Demux1/1 -> Divide/1
  Divide/1 -> Product/1

== system RLFactoryEnforceCrash6Opponents/RLServiceBOpponent/RLServiceAOpponentController/RLServiceEvasiveMoveChooser ==
  DiffRLX : Inport
  DiffRLY : Inport  Port=2
  DiffGoalX : Inport  Port=3
  DiffGoalY : Inport  Port=4
  Abs : Abs
  Abs1 : Abs
  Demux{,2..4} (4 alike) : Demux  Outputs=2
  Gain : Gain  Gain=-1
  Gain1 : Gain  Gain=-1
  Mux1 : Mux  Inputs=2
  Mux2 : Mux  Inputs=2
  Mux3 : Mux  Inputs=2
  Sqrt : Sqrt  SaturateOnIntegerOverflow=on
  Sqrt1 : Sqrt  SaturateOnIntegerOverflow=on
  Sum{,1..2,5} (4 alike) : Sum  Inputs=+|+
  Sum6 : Sum  Inputs=+|-
  Switch : Switch  Criteria=u2 > Threshold
  Switch1 : Switch  Criteria=u2 > Threshold
  EMX : Outport
  EMY : Outport  Port=2
  wires:
  Gain/1 -> Mux1/1
  DiffRLX/1 -> Gain1/1, Mux1/2
  Gain1/1 -> Mux2/2
  DiffGoalX/1 -> Mux3/1
  DiffGoalY/1 -> Mux3/2
  Mux3/1 -> Sum/2, Sum1/2
  Mux2/1 -> Sum/1, Demux4/1
  Mux1/1 -> Demux3/1, Sum1/1
  Sum1/1 -> Abs/1
  Sum/1 -> Abs1/1
  Abs1/1 -> Demux/1
  Demux/1 -> Sum2/1
  Demux/2 -> Sum2/2
  Demux2/2 -> Sum5/2
  Demux2/1 -> Sum5/1
  Abs/1 -> Demux2/1
  Sum5/1 -> Sqrt/1
  Sum2/1 -> Sqrt1/1
  Sqrt/1 -> Sum6/1
  Sqrt1/1 -> Sum6/2
  Sum6/1 -> Switch/2, Switch1/2
  Demux3/1 -> Switch/1
  Demux3/2 -> Switch1/1
  Demux4/1 -> Switch/3
  Demux4/2 -> Switch1/3
  Switch/1 -> EMX/1
  Switch1/1 -> EMY/1
  DiffRLY/1 -> Mux2/1, Gain/1

== system RLFactoryEnforceCrash6Opponents/RLServiceBOpponent/RLServiceAOpponentController/RLServiceInvalidMoveChecker ==
  MoveX : Inport
  MoveY : Inport  Port=2
  DiffRLX : Inport  Port=3
  DiffRLY : Inport  Port=4
  THRESHOLD : Inport  Port=5
  Constant5 : Constant
  Constant6 : Constant  Value=0
  Constant7 : Constant  Value=0
  Constant8 : Constant
  Constant9 : Constant
  Product : Product
  Product1 : Product
  Square : Math  Operator=square  SaturateOnIntegerOverflow=on
  Square Root : Sqrt  SaturateOnIntegerOverflow=on
  Square1 : Math  Operator=square  SaturateOnIntegerOverflow=on
  Sum : Sum  Inputs=+|-
  Sum1 : Sum
  Sum5 : Sum  Inputs=+|+
  Sum6 : Sum  Inputs=+|-|+
  Switch1 : Switch  Criteria=u2 > Threshold
  Switch3 : Switch  Criteria=u2 > Threshold
  MoveInValid : Outport
  wires:
  Product1/1 -> Sum5/2
  Sum5/1 -> Switch3/2
  Product/1 -> Sum5/1
  Sum6/1 -> MoveInValid/1
  Switch3/1 -> Sum6/1
  Constant9/1 -> Switch3/1
  MoveY/1 -> Product1/1
  MoveX/1 -> Product/1
  Constant8/1 -> Sum6/2
  Constant7/1 -> Switch3/3
  THRESHOLD/1 -> Sum/2
  Sum/1 -> Switch1/2
  Constant5/1 -> Switch1/3
  Constant6/1 -> Switch1/1
  Switch1/1 -> Sum6/3
  DiffRLY/1 -> Square1/1, Product1/2
  DiffRLX/1 -> Product/2, Square/1
  Square1/1 -> Sum1/2
  Sum1/1 -> Square Root/1
  Square/1 -> Sum1/1
  Square Root/1 -> Sum/1

== system RLFactoryEnforceCrash6Opponents/RLServiceBOpponent/RLServiceAOpponentController/RLServicePMAdjustVelocity ==
  MoveX : Inport
  MoveY : Inport  Port=2
  Velocity : Inport  Port=3
  Constant : Constant
  Demux1 : Demux  Outputs=2
  Divide : Product  Inputs=*/
  Divide1 : Product  Inputs=*/
  Mux : Mux  Inputs=2
  Product : Product
  Product3 : Product
  Sqrt1 : Sqrt  SaturateOnIntegerOverflow=on
  Square : Math  Operator=square  SaturateOnIntegerOverflow=on
  Square1 : Math  Operator=square  SaturateOnIntegerOverflow=on
  Sum : Sum  Inputs=+|+
  Switch : Switch  Criteria=u2 > Threshold
  AdjX : Outport
  AdjY : Outport  Port=2
  wires:
  Velocity/1 -> Product/2, Product3/2
  MoveX/1 -> Square/1, Mux/1
  MoveY/1 -> Square1/1, Mux/2
  Divide1/1 -> Product3/1
  Divide/1 -> Product/1
  Switch/1 -> Divide1/2, Divide/2
  Constant/1 -> Switch/3
  Mux/1 -> Demux1/1
  Demux1/2 -> Divide1/1
  Square1/1 -> Sum/2
  Sum/1 -> Sqrt1/1
  Demux1/1 -> Divide/1
  Product/1 -> AdjX/1
  Sqrt1/1 -> Switch/2, Switch/1
  Product3/1 -> AdjY/1
  Square/1 -> Sum/1

== system RLFactoryEnforceCrash6Opponents/RLServiceBOpponent/RLServiceAOpponentController/RLServiceXAvoidOvershooting ==
  MoveX : Inport
  MoveY : Inport  Port=2
  DiffToGoalX : Inport  Port=3
  DiffToGoalY : Inport  Port=4
  TS : Inport  Port=5
  Abs{1..4} (4 alike) : Abs
  Divide : Product  Inputs=*/
  Divide1 : Product  Inputs=*/
  Product : Product
  Product1 : Product
  Sum1 : Sum  Inputs=-|+
  Sum2 : Sum  Inputs=-|+
  Switch : Switch  Criteria=u2 > Threshold
  Switch1 : Switch  Criteria=u2 > Threshold
  MoveXNoOvershoot : Outport
  MoveYNoOvershoot : Outport  Port=2
  wires:
  Abs1/1 -> Sum1/2
  Switch/1 -> MoveXNoOvershoot/1
  Product/1 -> Abs2/1
  Abs2/1 -> Sum1/1
  DiffToGoalX/1 -> Divide/1, Abs1/1
  Sum1/1 -> Switch/2
  MoveX/1 -> Product/1, Switch/1
  Divide/1 -> Switch/3
  MoveY/1 -> Product1/1, Switch1/1
  Sum2/1 -> Switch1/2
  Abs4/1 -> Sum2/1
  Product1/1 -> Abs4/1
  Divide1/1 -> Switch1/3
  TS/1 -> Divide1/2, Product1/2, Divide/2, Product/2
  Abs3/1 -> Sum2/2
  Switch1/1 -> MoveYNoOvershoot/1
  DiffToGoalY/1 -> Divide1/1, Abs3/1

== system RLFactoryEnforceCrash6Opponents/RLServiceCOpponent/RLServiceAOpponentController/RLServiceArrivedChecker ==
  X : Inport
  Y : Inport  Port=2
  GoalX : Inport  Port=3
  GoalY : Inport  Port=4
  RLX : Inport  Port=5
  RLY : Inport  Port=6
  THRESHOLD : Inport  Port=7
  Constant1 : Constant
  Constant3 : Constant
  Constant4 : Constant  Value=0
  Constant5 : Constant  Value=0
  Constant6 : Constant
  Constant8 : Constant  Value=-BLOCKEDTIMER
  Integrator : Integrator  LimitOutput=on  UpperSaturationLimit=BLOCKEDTIMER  LowerSaturationLimit=0
  RLServiceEuclideanDistanceCalculator1 : Subsystem
  RLServiceEuclideanDistanceCalculator2 : Subsystem
  Sum : Sum  Inputs=|++
  Sum1 : Sum  Inputs=+-|
  Switch1 : Switch  Criteria=u2 > Threshold  Threshold=0.5
  Switch3 : Switch  Threshold=BLOCKEDTIMER
  Switch4 : Switch  Criteria=u2 > Threshold
  ArrivedCheck : Outport
  wires:
  RLServiceEuclideanDistanceCalculator1/1(DistToGoal) -> Switch1/2
  X/1 -> RLServiceEuclideanDistanceCalculator1/1(X)
  Switch1/1 -> Sum/1
  Constant3/1 -> Switch1/3
  Y/1 -> RLServiceEuclideanDistanceCalculator1/2(Y)
  Constant4/1 -> Switch1/1
  Sum/1 -> ArrivedCheck/1
  Switch3/1 -> Sum/2
  Integrator/1 -> Switch3/2
  Constant5/1 -> Switch3/3
  RLX/1 -> RLServiceEuclideanDistanceCalculator2/1(X)
  RLY/1 -> RLServiceEuclideanDistanceCalculator2/2(Y)
  GoalX/1 -> RLServiceEuclideanDistanceCalculator2/3(GoalX), RLServiceEuclideanDistanceCalculator1/3(GoalX)
  GoalY/1 -> RLServiceEuclideanDistanceCalculator2/4(GoalY), RLServiceEuclideanDistanceCalculator1/4(GoalY)
  RLServiceEuclideanDistanceCalculator2/1(OppDistToGoal) -> Sum1/1
  Constant8/1 -> Switch4/1
  Constant6/1 -> Switch4/3
  THRESHOLD/1 -> Sum1/2
  Sum1/1 -> Switch4/2
  Switch4/1 -> Integrator/1
  Constant1/1 -> Switch3/1

== system RLFactoryEnforceCrash6Opponents/RLServiceCOpponent/RLServiceAOpponentController/RLServiceEMAdjustVelocity ==
  MoveX : Inport
  MoveY : Inport  Port=2
  Velocity : Inport  Port=3
  Constant : Constant
  Demux1 : Demux  Outputs=2
  Divide : Product  Inputs=*/
  Divide1 : Product  Inputs=*/
  Mux : Mux  Inputs=2
  Product : Product
  Product3 : Product
  Sqrt1 : Sqrt  SaturateOnIntegerOverflow=on
  Square : Math  Operator=square  SaturateOnIntegerOverflow=on
  Square1 : Math  Operator=square  SaturateOnIntegerOverflow=on
  Sum : Sum  Inputs=+|+
  Switch : Switch  Criteria=u2 > Threshold
  AdjX : Outport
  AdjY : Outport  Port=2
  wires:
  Product/1 -> AdjX/1
  MoveY/1 -> Square1/1, Mux/2
  Mux/1 -> Demux1/1
  Divide1/1 -> Product3/1
  Constant/1 -> Switch/3
  Square1/1 -> Sum/2
  Switch/1 -> Divide1/2, Divide/2
  Velocity/1 -> Product/2, Product3/2
  Sum/1 -> Sqrt1/1
  Square/1 -> Sum/1
  Sqrt1/1 -> Switch/2, Switch/1
  Product3/1 -> AdjY/1
  Demux1/2 -> Divide1/1
  MoveX/1 -> Square/1, Mux/1
  Demux1/1 -> Divide/1
  Divide/1 -> Product/1

== system RLFactoryEnforceCrash6Opponents/RLServiceCOpponent/RLServiceAOpponentController/RLServiceEvasiveMoveChooser ==
  DiffRLX : Inport
  DiffRLY : Inport  Port=2
  DiffGoalX : Inport  Port=3
  DiffGoalY : Inport  Port=4
  Abs : Abs
  Abs1 : Abs
  Demux{,2..4} (4 alike) : Demux  Outputs=2
  Gain : Gain  Gain=-1
  Gain1 : Gain  Gain=-1
  Mux1 : Mux  Inputs=2
  Mux2 : Mux  Inputs=2
  Mux3 : Mux  Inputs=2
  Sqrt : Sqrt  SaturateOnIntegerOverflow=on
  Sqrt1 : Sqrt  SaturateOnIntegerOverflow=on
  Sum{,1..2,5} (4 alike) : Sum  Inputs=+|+
  Sum6 : Sum  Inputs=+|-
  Switch : Switch  Criteria=u2 > Threshold
  Switch1 : Switch  Criteria=u2 > Threshold
  EMX : Outport
  EMY : Outport  Port=2
  wires:
  Gain/1 -> Mux1/1
  DiffRLX/1 -> Gain1/1, Mux1/2
  Gain1/1 -> Mux2/2
  DiffGoalX/1 -> Mux3/1
  DiffGoalY/1 -> Mux3/2
  Mux3/1 -> Sum/2, Sum1/2
  Mux2/1 -> Sum/1, Demux4/1
  Mux1/1 -> Demux3/1, Sum1/1
  Sum1/1 -> Abs/1
  Sum/1 -> Abs1/1
  Abs1/1 -> Demux/1
  Demux/1 -> Sum2/1
  Demux/2 -> Sum2/2
  Demux2/2 -> Sum5/2
  Demux2/1 -> Sum5/1
  Abs/1 -> Demux2/1
  Sum5/1 -> Sqrt/1
  Sum2/1 -> Sqrt1/1
  Sqrt/1 -> Sum6/1
  Sqrt1/1 -> Sum6/2
  Sum6/1 -> Switch/2, Switch1/2
  Demux3/1 -> Switch/1
  Demux3/2 -> Switch1/1
  Demux4/1 -> Switch/3
  Demux4/2 -> Switch1/3
  Switch/1 -> EMX/1
  Switch1/1 -> EMY/1
  DiffRLY/1 -> Mux2/1, Gain/1

== system RLFactoryEnforceCrash6Opponents/RLServiceCOpponent/RLServiceAOpponentController/RLServiceInvalidMoveChecker ==
  MoveX : Inport
  MoveY : Inport  Port=2
  DiffRLX : Inport  Port=3
  DiffRLY : Inport  Port=4
  THRESHOLD : Inport  Port=5
  Constant5 : Constant
  Constant6 : Constant  Value=0
  Constant7 : Constant  Value=0
  Constant8 : Constant
  Constant9 : Constant
  Product : Product
  Product1 : Product
  Square : Math  Operator=square  SaturateOnIntegerOverflow=on
  Square Root : Sqrt  SaturateOnIntegerOverflow=on
  Square1 : Math  Operator=square  SaturateOnIntegerOverflow=on
  Sum : Sum  Inputs=+|-
  Sum1 : Sum
  Sum5 : Sum  Inputs=+|+
  Sum6 : Sum  Inputs=+|-|+
  Switch1 : Switch  Criteria=u2 > Threshold
  Switch3 : Switch  Criteria=u2 > Threshold
  MoveInValid : Outport
  wires:
  Product1/1 -> Sum5/2
  Sum5/1 -> Switch3/2
  Product/1 -> Sum5/1
  Sum6/1 -> MoveInValid/1
  Switch3/1 -> Sum6/1
  Constant9/1 -> Switch3/1
  MoveY/1 -> Product1/1
  MoveX/1 -> Product/1
  Constant8/1 -> Sum6/2
  Constant7/1 -> Switch3/3
  THRESHOLD/1 -> Sum/2
  Sum/1 -> Switch1/2
  Constant5/1 -> Switch1/3
  Constant6/1 -> Switch1/1
  Switch1/1 -> Sum6/3
  DiffRLY/1 -> Square1/1, Product1/2
  DiffRLX/1 -> Product/2, Square/1
  Square1/1 -> Sum1/2
  Sum1/1 -> Square Root/1
  Square/1 -> Sum1/1
  Square Root/1 -> Sum/1

== system RLFactoryEnforceCrash6Opponents/RLServiceCOpponent/RLServiceAOpponentController/RLServicePMAdjustVelocity ==
  MoveX : Inport
  MoveY : Inport  Port=2
  Velocity : Inport  Port=3
  Constant : Constant
  Demux1 : Demux  Outputs=2
  Divide : Product  Inputs=*/
  Divide1 : Product  Inputs=*/
  Mux : Mux  Inputs=2
  Product : Product
  Product3 : Product
  Sqrt1 : Sqrt  SaturateOnIntegerOverflow=on
  Square : Math  Operator=square  SaturateOnIntegerOverflow=on
  Square1 : Math  Operator=square  SaturateOnIntegerOverflow=on
  Sum : Sum  Inputs=+|+
  Switch : Switch  Criteria=u2 > Threshold
  AdjX : Outport
  AdjY : Outport  Port=2
  wires:
  Velocity/1 -> Product/2, Product3/2
  MoveX/1 -> Square/1, Mux/1
  MoveY/1 -> Square1/1, Mux/2
  Divide1/1 -> Product3/1
  Divide/1 -> Product/1
  Switch/1 -> Divide1/2, Divide/2
  Constant/1 -> Switch/3
  Mux/1 -> Demux1/1
  Demux1/2 -> Divide1/1
  Square1/1 -> Sum/2
  Sum/1 -> Sqrt1/1
  Demux1/1 -> Divide/1
  Product/1 -> AdjX/1
  Sqrt1/1 -> Switch/2, Switch/1
  Product3/1 -> AdjY/1
  Square/1 -> Sum/1

== system RLFactoryEnforceCrash6Opponents/RLServiceCOpponent/RLServiceAOpponentController/RLServiceXAvoidOvershooting ==
  MoveX : Inport
  MoveY : Inport  Port=2
  DiffToGoalX : Inport  Port=3
  DiffToGoalY : Inport  Port=4
  TS : Inport  Port=5
  Abs{1..4} (4 alike) : Abs
  Divide : Product  Inputs=*/
  Divide1 : Product  Inputs=*/
  Product : Product
  Product1 : Product
  Sum1 : Sum  Inputs=-|+
  Sum2 : Sum  Inputs=-|+
  Switch : Switch  Criteria=u2 > Threshold
  Switch1 : Switch  Criteria=u2 > Threshold
  MoveXNoOvershoot : Outport
  MoveYNoOvershoot : Outport  Port=2
  wires:
  Abs1/1 -> Sum1/2
  Switch/1 -> MoveXNoOvershoot/1
  Product/1 -> Abs2/1
  Abs2/1 -> Sum1/1
  DiffToGoalX/1 -> Divide/1, Abs1/1
  Sum1/1 -> Switch/2
  MoveX/1 -> Product/1, Switch/1
  Divide/1 -> Switch/3
  MoveY/1 -> Product1/1, Switch1/1
  Sum2/1 -> Switch1/2
  Abs4/1 -> Sum2/1
  Product1/1 -> Abs4/1
  Divide1/1 -> Switch1/3
  TS/1 -> Divide1/2, Product1/2, Divide/2, Product/2
  Abs3/1 -> Sum2/2
  Switch1/1 -> MoveYNoOvershoot/1
  DiffToGoalY/1 -> Divide1/1, Abs3/1

== system RLFactoryEnforceCrash6Opponents/RLServiceDOpponent/RLServiceAOpponentController/RLServiceArrivedChecker ==
  X : Inport
  Y : Inport  Port=2
  GoalX : Inport  Port=3
  GoalY : Inport  Port=4
  RLX : Inport  Port=5
  RLY : Inport  Port=6
  THRESHOLD : Inport  Port=7
  Constant1 : Constant
  Constant3 : Constant
  Constant4 : Constant  Value=0
  Constant5 : Constant  Value=0
  Constant6 : Constant
  Constant8 : Constant  Value=-BLOCKEDTIMER
  Integrator : Integrator  LimitOutput=on  UpperSaturationLimit=BLOCKEDTIMER  LowerSaturationLimit=0
  RLServiceEuclideanDistanceCalculator1 : Subsystem
  RLServiceEuclideanDistanceCalculator2 : Subsystem
  Sum : Sum  Inputs=|++
  Sum1 : Sum  Inputs=+-|
  Switch1 : Switch  Criteria=u2 > Threshold  Threshold=0.5
  Switch3 : Switch  Threshold=BLOCKEDTIMER
  Switch4 : Switch  Criteria=u2 > Threshold
  ArrivedCheck : Outport
  wires:
  RLServiceEuclideanDistanceCalculator1/1(DistToGoal) -> Switch1/2
  X/1 -> RLServiceEuclideanDistanceCalculator1/1(X)
  Switch1/1 -> Sum/1
  Constant3/1 -> Switch1/3
  Y/1 -> RLServiceEuclideanDistanceCalculator1/2(Y)
  Constant4/1 -> Switch1/1
  Sum/1 -> ArrivedCheck/1
  Switch3/1 -> Sum/2
  Integrator/1 -> Switch3/2
  Constant5/1 -> Switch3/3
  RLX/1 -> RLServiceEuclideanDistanceCalculator2/1(X)
  RLY/1 -> RLServiceEuclideanDistanceCalculator2/2(Y)
  GoalX/1 -> RLServiceEuclideanDistanceCalculator2/3(GoalX), RLServiceEuclideanDistanceCalculator1/3(GoalX)
  GoalY/1 -> RLServiceEuclideanDistanceCalculator2/4(GoalY), RLServiceEuclideanDistanceCalculator1/4(GoalY)
  RLServiceEuclideanDistanceCalculator2/1(OppDistToGoal) -> Sum1/1
  Constant8/1 -> Switch4/1
  Constant6/1 -> Switch4/3
  THRESHOLD/1 -> Sum1/2
  Sum1/1 -> Switch4/2
  Switch4/1 -> Integrator/1
  Constant1/1 -> Switch3/1

== system RLFactoryEnforceCrash6Opponents/RLServiceDOpponent/RLServiceAOpponentController/RLServiceEMAdjustVelocity ==
  MoveX : Inport
  MoveY : Inport  Port=2
  Velocity : Inport  Port=3
  Constant : Constant
  Demux1 : Demux  Outputs=2
  Divide : Product  Inputs=*/
  Divide1 : Product  Inputs=*/
  Mux : Mux  Inputs=2
  Product : Product
  Product3 : Product
  Sqrt1 : Sqrt  SaturateOnIntegerOverflow=on
  Square : Math  Operator=square  SaturateOnIntegerOverflow=on
  Square1 : Math  Operator=square  SaturateOnIntegerOverflow=on
  Sum : Sum  Inputs=+|+
  Switch : Switch  Criteria=u2 > Threshold
  AdjX : Outport
  AdjY : Outport  Port=2
  wires:
  Product/1 -> AdjX/1
  MoveY/1 -> Square1/1, Mux/2
  Mux/1 -> Demux1/1
  Divide1/1 -> Product3/1
  Constant/1 -> Switch/3
  Square1/1 -> Sum/2
  Switch/1 -> Divide1/2, Divide/2
  Velocity/1 -> Product/2, Product3/2
  Sum/1 -> Sqrt1/1
  Square/1 -> Sum/1
  Sqrt1/1 -> Switch/2, Switch/1
  Product3/1 -> AdjY/1
  Demux1/2 -> Divide1/1
  MoveX/1 -> Square/1, Mux/1
  Demux1/1 -> Divide/1
  Divide/1 -> Product/1

== system RLFactoryEnforceCrash6Opponents/RLServiceDOpponent/RLServiceAOpponentController/RLServiceEvasiveMoveChooser ==
  DiffRLX : Inport
  DiffRLY : Inport  Port=2
  DiffGoalX : Inport  Port=3
  DiffGoalY : Inport  Port=4
  Abs : Abs
  Abs1 : Abs
  Demux{,2..4} (4 alike) : Demux  Outputs=2
  Gain : Gain  Gain=-1
  Gain1 : Gain  Gain=-1
  Mux1 : Mux  Inputs=2
  Mux2 : Mux  Inputs=2
  Mux3 : Mux  Inputs=2
  Sqrt : Sqrt  SaturateOnIntegerOverflow=on
  Sqrt1 : Sqrt  SaturateOnIntegerOverflow=on
  Sum{,1..2,5} (4 alike) : Sum  Inputs=+|+
  Sum6 : Sum  Inputs=+|-
  Switch : Switch  Criteria=u2 > Threshold
  Switch1 : Switch  Criteria=u2 > Threshold
  EMX : Outport
  EMY : Outport  Port=2
  wires:
  Gain/1 -> Mux1/1
  DiffRLX/1 -> Gain1/1, Mux1/2
  Gain1/1 -> Mux2/2
  DiffGoalX/1 -> Mux3/1
  DiffGoalY/1 -> Mux3/2
  Mux3/1 -> Sum/2, Sum1/2
  Mux2/1 -> Sum/1, Demux4/1
  Mux1/1 -> Demux3/1, Sum1/1
  Sum1/1 -> Abs/1
  Sum/1 -> Abs1/1
  Abs1/1 -> Demux/1
  Demux/1 -> Sum2/1
  Demux/2 -> Sum2/2
  Demux2/2 -> Sum5/2
  Demux2/1 -> Sum5/1
  Abs/1 -> Demux2/1
  Sum5/1 -> Sqrt/1
  Sum2/1 -> Sqrt1/1
  Sqrt/1 -> Sum6/1
  Sqrt1/1 -> Sum6/2
  Sum6/1 -> Switch/2, Switch1/2
  Demux3/1 -> Switch/1
  Demux3/2 -> Switch1/1
  Demux4/1 -> Switch/3
  Demux4/2 -> Switch1/3
  Switch/1 -> EMX/1
  Switch1/1 -> EMY/1
  DiffRLY/1 -> Mux2/1, Gain/1
